simulink model "path_finder"  (Simulink 8.7)
settings: Solver=FixedStepAuto  StartTime=0.0  StopTime=10.0  FixedStep=0.01  RelTol=1e-3
undefined symbols (not defined in the file or in its folder): get, hot
libraries: dspsnks4 x1
settings Model: Creator=eispin  LastModifiedBy=eispin
settings DataIOCC: LimitDataPoints=off  SaveFormat=Dataset
settings DebuggingCC: UnderspecifiedInitializationDetection=Simplified  MergeDetectMultiDrivingBlocksExec=error
settings HardwareCC: ProdBitPerPointer=64  ProdLargestAtomicFloat=Float  ProdIntDivRoundTo=Zero  ProdEndianess=LittleEndian  ProdWordSize=64  ProdHWDeviceType=Intel->x86-64 (Windows64)
settings ModelReferenceCC: PropagateSignalLabelsOutOfModel=on
settings ConfigComp: CovModelRefEnable=off

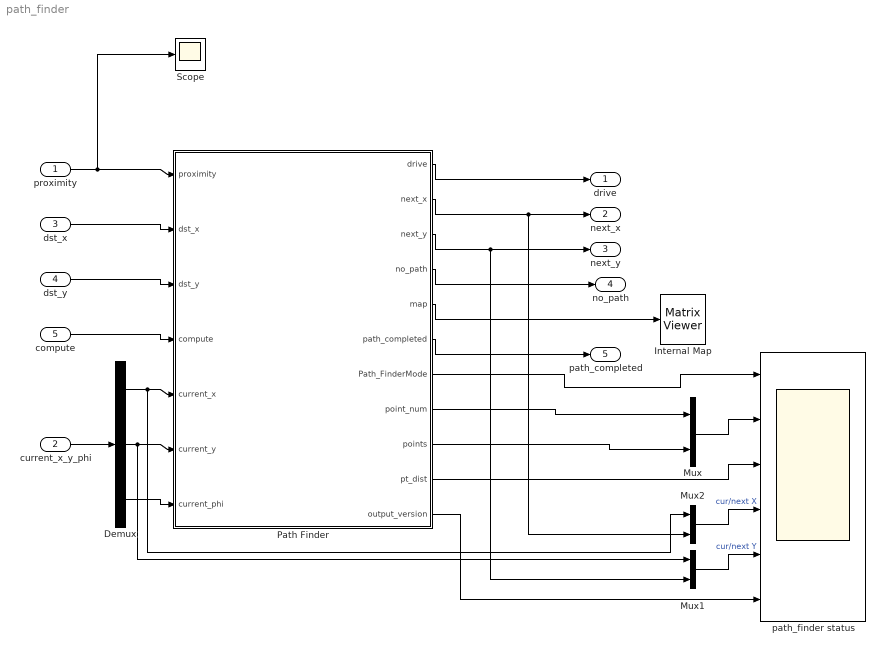
== system path_finder ==
  proximity : Inport  PortDimensions=[8]
  current_x_y_phi : Inport  Port=2  PortDimensions=[3]
  dst_x : Inport  Port=3
  dst_y : Inport  Port=4
  compute : Inport  Port=5
  Demux : Demux  Outputs=3
  Internal Map : dspsnks4/Matrix Viewer  ImageParams=off  CMapStr=hot(256)  AxisColorbar=off  AxisParams=off  AxisOrigin=Lower left corner  AxisTickMode=Auto  XTickRange=[0 1]  YTickRange=[0 1]  XLabel=X-axis  YLabel=Y-axis  ZLabel=Z-axis  FigPos=get(0,'defaultfigureposition')  AxisZoom=off
      settings: YMin=0  YMax=1
  Mux : Mux  Inputs=2
  Mux1 : Mux  Inputs=2
  Mux2 : Mux  Inputs=2
  Path Finder : Stateflow chart  TreatAsAtomicUnit=on
  Scope : Scope
  path_finder status : Scope  NumInputPorts=6
  drive : Outport
  next_x : Outport  Port=2
  next_y : Outport  Port=3
  no_path : Outport  Port=4
  path_completed : Outport  Port=5
  wires:
  proximity/1 -> Scope/1, Path Finder/1(proximity)
  dst_x/1 -> Path Finder/2(dst_x)
  dst_y/1 -> Path Finder/3(dst_y)
  compute/1 -> Path Finder/4(compute)
  Path Finder/1(drive) -> drive/1
  Path Finder/2(next_x) -> Mux2/2, next_x/1
  Path Finder/3(next_y) -> Mux1/2, next_y/1
  Path Finder/4(no_path) -> no_path/1
  Path Finder/5(map) -> Internal Map/1
  current_x_y_phi/1 -> Demux/1
  Demux/1 -> Mux2/1, Path Finder/5(current_x)
  Demux/2 -> Mux1/1, Path Finder/6(current_y)
  Demux/3 -> Path Finder/7(current_phi)
  Path Finder/6(path_completed) -> path_completed/1
  Path Finder/7(Path_FinderMode) -> path_finder status/1
  Path Finder/8(point_num) -> Mux/1
  Path Finder/9(points) -> Mux/2
  Mux/1 -> path_finder status/2
  Path Finder/10(pt_dist) -> path_finder status/3
  Mux2/1 -> path_finder status/4  "cur/next X"
  Mux1/1 -> path_finder status/5  "cur/next Y"
  Path Finder/11(output_version) -> path_finder status/6

== stateflow chart Path Finder ==
  state Collecting
    during:
    for i = 1:8
    [r, c] = calculate_cell(proximity(i) + 2.5, current_phi + VIEW_DIRECTIONS(i));
    if (r ~= -1)
    map(rows + 1 - r, c) = 1;
    end
    end
    state Inactive
    state Running
      entry:
      next_x = current_x;
      next_y = current_y;
      during:
      coder.extrinsic('TinUtils.get_path_point');
      if point_num <= points
      pt_dist = norm([current_x-next_x; current_y-next_y]);
      if  pt_dist <= drive_tolerance
      point_num = point_num + 1
      drive = 0;
      next_x = TinUtils.convert_path_point(TinUtils.get_path_point(path, point_num, 1));
      next_y = TinUtils.convert_path_point(TinUtils.get_path_point(path, point_num, 2));
      output_version = output_version + 1;
      else
      step_phi = atan2(next_y - current_y, next_x - current_x);
      drive = 1;
      end
      end
      ex:
      drive = 0;
    state WaitZero
      ex:
      path_completed = 0;
      no_path = 0;
    state ComputePath
      en:
      coder.extrinsic('TinUtils.calculate_path');
      path = TinUtils.calculate_path(map, dst_x, dst_y, current_x, current_y);
      points = TinUtils.get_path_length(path);
      if isempty(path)
      no_path = 1;
      end
      point_num = 1;
    (default) -> Inactive
    WaitZero -> Inactive : [compute == 0]
    Inactive -> ComputePath : [compute == 1] {
        | 	coder.extrinsic('TinUtils.calculate_path');
        | 	path = TinUtils.calculate_path(map, dst_x, dst_y, current_x, current_y);
        | 	points = TinUtils.get_path_length(path);
        | }
    Running -> WaitZero [order 1] : [point_num > points]{path_completed = 1;}
    ComputePath -> WaitZero [order 1] : [no_path ~= 0]
    ComputePath -> Running [order 2] : [no_path == 0]
    Running -> ComputePath [order 2] : [drive == 1 && path_blocked() == 1]
  note: Precisely the following variables contain
      | coordinates which is "mirrored":
      | - map
  (default) -> Collecting : {
      | 	% write initial variables
      | 	drive = 0;
      | 	next_x = 0;
      | 	next_y = 0;
      | 	no_path = 0;
      | 	% sensor view directions from:
      | 	% https:%www.cyberbotics.com/guide/using-the-e-puck-robot.php
      | 	VIEW_DIRECTIONS = [mod(1.27 - pi/2, 2 * pi)     mod(0.77 - pi/2, 2 * pi)     mod(0.00 - pi/2, 2 * pi)    mod(5.21 - pi/2, 2 * pi) ...
      |                                             mod(4.21 - pi/2, 2 * pi)     mod(pi - pi/2, 2 * pi)          mod(2.37 - pi/2, 2 * pi)    mod(1.87 - pi/2, 2 * pi)];
      | 	% create 200x200 matrix filled with zeros
      | 	map = zeros(rows, cols);
      | }
  data: distance function_input double; direction function_input double; row function_output double; col function_output double; is_blocked function_output double; drive output double; proximity input double size=8; dst_x input double; dst_y input double; next_x output double; next_y output double; compute input double; no_path output double; map output double; current_x input double; current_y input double; r local double; c local double; VIEW_DIRECTIONS local double; current_phi input double; path local double; path_completed output double; cols constant double =200; rows constant double =200; step_phi local double; Path_FinderMode output Enum: Path_FinderModeType1; point_num output double; points output double =0; i local double; drive_tolerance constant double =0.7; pt_dist output double; output_version output double =0
  function [row, col] = calculate_cell(distance, direction):
    | function [row, col] = calculate_cell(distance, direction)
    |     row = floor(current_y + distance * sin(direction));
    |     col = floor(current_x + distance * cos(direction));
    |     if ~TinUtils.is_inside([row col], rows, cols)
    |         row = -1;
    |         col = -1;
    |     end
    | end
  function is_blocked = path_blocked:
    | function is_blocked = path_blocked()
    | 
    | % Can't easily use IR sensors here, since path_executor rotates around a
    | % lot.
    | 
    | r = floor(current_y);
    | c = floor(current_x);
    | % Must "forwards-mirror" the input (r,c,phi), which is "unmirrored" data
    | [drivable_distance, ~] = TinUtils.raycast_polymorphic(map, rows + 1 - r, c, -step_phi, 5);
    |     % Choosing '50' has the side-effect that we first run up to the wall
    |     % before noticing that there *is* one.
    |     % and only then try 
    | % "Unmirroring" the distance is no-op
    | drivable_distance = drivable_distance + TinUtils.radius;
    | expect_distance = norm([next_x next_y] - [current_x current_y]);
    | 
    | is_blocked = expect_distance > drivable_distance + drive_tolerance;
    | 
    | end
